simulink model "ssc_auto_ev_20b"  (R2020b)
settings: Solver=VariableStepAuto  StartTime=0.0  StopTime=200  RelTol=1e-3  AbsTol=1e-3
PreLoadFcn:
  | % Simulation parameters
  | dt = 0.01;
  | 
  | % Battery cell parameters
  | ssc_lithium_cell_1RC_ini
  | Nseries = 100;
  | Nparallel = 10;
  | 
  | % Motor parameters
  | max_torque = 220;
  | max_power = 80e3;
  | 
  | % Vehicle parameters
  | vehicle_mass = 4000;
  | wheel_radius = 0.35;
  | area = 5;
  | drag_coefficient = 0.25;
  | air_density = 1.225;
  | gravity = 9.81;
  | rolling_res_ratio = 0.015;
  | 
  | % Differential drive parameters
  | gear_ratio = 12;
  | 
  | % Simplified braking system parameters
  | force_max_pedal = 500;
  | braking_torque_to_pedal_force_ratio = -16;
  | 
  | % Vehicle controller parameters
  | hill_hold_max_speed = 0.5;
  | 
  | % Water properties for cooling circuit
  | load WaterProperties
  | 
  | % Input signals for Signal Editor block
  | load ssc_auto_ev_Inputs
values from neighbouring files (symbols this model uses):
  C1_LUT = [1913.6 4625.7 23306 10736 18036 12251 9022.9 12447 18872 40764 18721 33630 ... (21 elements, 7x3)]    [ssc_auto_ev_param.mat]
  Capacity_LUT = [28.0081 27.625 27.6392]    [ssc_auto_ev_param.mat]
  cell_Cp_heat = 810.5328    [ssc_auto_ev_param.mat]
  cell_mass = 1    [ssc_auto_ev_param.mat]
  Em_LUT = [3.4966 3.5519 3.6183 3.7066 3.9131 4.0748 4.1923 3.5057 3.566 3.6337 3.7127 3.9259 ... (21 elements, 7x3)]    [ssc_auto_ev_param.mat]
  Qe_init = 15.6845    [ssc_auto_ev_param.mat]
  R0_LUT = [0.0117 0.011 0.0114 0.0107 0.0107 0.0113 0.0116 0.0085 0.0085 0.0087 0.0082 0.0083 ... (21 elements, 7x3)]    [ssc_auto_ev_param.mat]
  R1_LUT = [0.0109 0.0069 0.0047 0.0034 0.0033 0.0033 0.0028 0.0029 0.0024 0.0026 0.0016 0.0023 ... (21 elements, 7x3)]    [ssc_auto_ev_param.mat]
  SOC_LUT = [0 0.1 0.25 0.5 0.75 0.9 1]    [ssc_auto_ev_param.mat]
  T_init = 293.15    [ssc_auto_ev_param.mat]
  Temperature_LUT = [278.15 293.15 313.15]    [ssc_auto_ev_param.mat]
undefined symbols (not defined in the file or in its folder): DiscIntNeverNeededParam, K, Lambda, tau, x0
libraries: fl_lib x656, nesl_utility x86, simulink x21, LiBatteryElements_lib x16, SignalEditorBlockLib x4, simulink_extras x4
(part 3 of 13)

== system ssc_auto_ev_20b/Step 4: Deployment Model ==
  note: Turn on sample time colors to validate timing. To do this, from the
      | DEBUG->DIAGNOSTICS menu select Information Overlays->Colors.
  Battery @50Hz : Subsystem
      settings: PortSchema="{\"entries\":[{\"content\":{\"sides\":[{\"content\":{\"connectorIds\":[\"In1\",\"Out2\"]},\"type\":\"ConnectorPlacement.EquallySpacedRectSide\",\"uuid\":\"54b288da-0e57-4d78-b35e-d63e4748356c\"},{\"content\":{\"connectorIds\":[\"Out1\",\"In2\"],\"side\":\"RIGHT\"},\"type\":\"ConnectorPlacement.EquallySpacedRectSide\",\"uuid\":\"06deb6c0-981d-4564-ae11-64776ad4ca27\"},{\"content\":{\"connectorIds\":[],\"side\":\"TOP\"},\"type\":\"ConnectorPlacement.EquallySpacedRectSide\",\"uuid\":\"0b8fba6d-2ee9-459b-aee7-2e2793598ae9\"}]},\"type\":\"ConnectorPlacement.EquallySpacedConnector\",\"uuid\":\"3f5b1629-deda-4b64-ac52-f3df4bebf2e4\"}],\"packageUris\":[\"http://schema.mathworks.com/mf0/Connector/R2020b\"],\"version\":\"1.0\"}"
  Control @100Hz : Subsystem
      settings: PortSchema="{\"entries\":[{\"content\":{\"sides\":[{\"content\":{\"connectorIds\":[]},\"type\":\"ConnectorPlacement.EquallySpacedRectSide\",\"uuid\":\"ef87f14a-ebef-48e8-8256-297aaa1e6a9a\"},{\"content\":{\"connectorIds\":[\"Out1\",\"In1\",\"Out2\",\"Out3\"],\"side\":\"RIGHT\"},\"type\":\"ConnectorPlacement.EquallySpacedRectSide\",\"uuid\":\"2f0c5370-6858-4894-ab47-0af24eaee6ce\"},{\"content\":{\"connectorIds\":[],\"side\":\"TOP\"},\"type\":\"ConnectorPlacement.EquallySpacedRectSide\",\"uuid\":\"12af46f8-0356-4b52-aec4-5ed7dbf12bbb\"}]},\"type\":\"ConnectorPlacement.EquallySpacedConnector\",\"uuid\":\"d882ff77-9b94-4690-a03a-88e1ef90f3db\"}],\"packageUris\":[\"http://schema.mathworks.com/mf0/Connector/R2020b\"],\"version\":\"1.0\"}"
  Rate Transition{,1..3} (4 alike) : RateTransition
  Rate transition (fast-to-slow){,1..3} (4 alike) : RateTransition  Integrity=off
  Rate transition (slow-to-fast){,1..3} (4 alike) : RateTransition  Integrity=off
  Thermal @20Hz : Subsystem
      settings: PortSchema="{\"entries\":[{\"content\":{\"sides\":[{\"content\":{\"connectorIds\":[\"In1\"]},\"type\":\"ConnectorPlacement.EquallySpacedRectSide\",\"uuid\":\"720b38ef-f1a9-4b25-942c-9d80c372deb3\"},{\"content\":{\"connectorIds\":[\"Out1\",\"In2\",\"Out2\",\"In3\",\"Out3\",\"In4\"],\"side\":\"RIGHT\"},\"type\":\"ConnectorPlacement.EquallySpacedRectSide\",\"uuid\":\"5564f5e5-3aff-4d95-92a7-b7874cc9818e\"},{\"content\":{\"connectorIds\":[],\"side\":\"TOP\"},\"type\":\"ConnectorPlacement.EquallySpacedRectSide\",\"uuid\":\"b2c1fdb5-3bc7-4a17-8874-08ad49945e58\"}]},\"type\":\"ConnectorPlacement.EquallySpacedConnector\",\"uuid\":\"56dd2a05-31e7-46fe-9962-826aaa21137d\"}],\"packageUris\":[\"http://schema.mathworks.com/mf0/Connector/R2020b\"],\"version\":\"1.0\"}"
  Vehicle and drive @100Hz : Subsystem
      settings: PortSchema="{\"entries\":[{\"content\":{\"sides\":[{\"content\":{\"connectorIds\":[\"In1\",\"Out1\",\"In2\",\"In3\",\"Out2\",\"In4\",\"Out3\",\"In5\",\"Out4\"]},\"type\":\"ConnectorPlacement.EquallySpacedRectSide\",\"uuid\":\"f314639a-2b4d-4845-a867-9fc19a275e88\"},{\"content\":{\"connectorIds\":[],\"side\":\"RIGHT\"},\"type\":\"ConnectorPlacement.EquallySpacedRectSide\",\"uuid\":\"94dc3db5-d98f-4c0a-adac-a7539403b4cc\"},{\"content\":{\"connectorIds\":[],\"side\":\"TOP\"},\"type\":\"ConnectorPlacement.EquallySpacedRectSide\",\"uuid\":\"a0a136c3-fb8b-4f8b-b3eb-c92638fab684\"}]},\"type\":\"ConnectorPlacement.EquallySpacedConnector\",\"uuid\":\"37a7cf0b-d138-4d1f-ae2f-6d44546dc5a7\"}],\"packageUris\":[\"http://schema.mathworks.com/mf0/Connector/R2020b\"],\"version\":\"1.0\"}"
  wires:
  Rate Transition/1 -> Thermal @20Hz/1(T)
  Rate transition (fast-to-slow)/1 -> Thermal @20Hz/2(temperature)
  Rate transition (fast-to-slow)2/1 -> Thermal @20Hz/3(temperature1)
  Rate transition (fast-to-slow)1/1 -> Thermal @20Hz/4(temperature2)
  Thermal @20Hz/1(heat flow) -> Rate transition (slow-to-fast)/1
  Thermal @20Hz/2(heat flow1) -> Rate transition (slow-to-fast)2/1
  Thermal @20Hz/3(heat flow2) -> Rate transition (slow-to-fast)1/1
  Rate transition (slow-to-fast)/1 -> Battery @50Hz/1(heat flow)
  Rate transition (fast-to-slow)3/1 -> Battery @50Hz/2(current)
  Battery @50Hz/1(voltage) -> Rate transition (slow-to-fast)3/1
  Battery @50Hz/2(temperature) -> Rate transition (fast-to-slow)/1
  Rate Transition2/1 -> Vehicle and drive @100Hz/1(Test data)
  Rate Transition1/1 -> Vehicle and drive @100Hz/2(iRef)
  Rate transition (slow-to-fast)3/1 -> Vehicle and drive @100Hz/3(voltage)
  Rate transition (slow-to-fast)2/1 -> Vehicle and drive @100Hz/4(heat flow)
  Rate transition (slow-to-fast)1/1 -> Vehicle and drive @100Hz/5(heat flow1)
  Vehicle and drive @100Hz/1(w) -> Rate Transition3/1
  Vehicle and drive @100Hz/2(current) -> Rate transition (fast-to-slow)3/1
  Vehicle and drive @100Hz/3(temperature) -> Rate transition (fast-to-slow)2/1
  Vehicle and drive @100Hz/4(temperature1) -> Rate transition (fast-to-slow)1/1
  Rate Transition3/1 -> Control @100Hz/1(In1)
  Control @100Hz/1(Veh) -> Rate Transition2/1
  Control @100Hz/2(Out2) -> Rate Transition1/1
  Control @100Hz/3(Env) -> Rate Transition/1

== system ssc_auto_ev_20b/Vehicle Dynamics ==
  Test data : Inport
  Brake Torque : Subsystem
  Bus Selector : BusSelector  OutputSignals=Incline,Wind speed,Brake pedal
  Drag and Gravity : Subsystem
  Final Drive Ratio : fl_lib/Mechanical/Mechanisms/Gear Box  ratio=gear_ratio  t_in_specify=off  t_in_priority=High  t_in=0 N*m  t_in_nominal_specify=off  t_in_nominal_unit=N*m  t_in_nominal_value=1  t_out_specify=off  t_out_priority=High  t_out=0 N*m  t_out_nominal_specify=off  t_out_nominal_unit=N*m  t_out_nominal_value=1
      settings: SourceProductBaseCode=PW,SS,VE
  Force Source : fl_lib/Mechanical/Mechanical Sources/Ideal Force Source
      settings: SourceProductBaseCode=PW,SS,VE
  MTRef : fl_lib/Mechanical/Translational Elements/Mechanical Translational Reference
      settings: SourceProductBaseCode=PW,SS,VE
  PS Subtract : fl_lib/Physical Signals/Functions/PS Subtract
      settings: SourceProductBaseCode=PW,SS,VE
  Sensing Speed : Subsystem
      mask Display: disp('v')
  Vehicle Mass : fl_lib/Mechanical/Translational Elements/Mass  mass=vehicle_mass kg  num_ports=foundation.enum.numPorts2.one  v_specify=off  v_priority=High  v=0 m/s  v_nominal_specify=off  v_nominal_unit=m/s  v_nominal_value=1  f_specify=off  f_priority=High  f=0 N  f_nominal_specify=off  f_nominal_unit=N  f_nominal_value=1
      settings: SourceProductBaseCode=PW,SS,VE
  Wheel and Axle : fl_lib/Mechanical/Mechanisms/Wheel and Axle  R=wheel_radius m  or=1  t_specify=off  t_priority=High  t=0 N*m  t_nominal_specify=off  t_nominal_unit=N*m  t_nominal_value=1  f_specify=off  f_priority=High  f=0 N  f_nominal_specify=off  f_nominal_unit=N  f_nominal_value=1
      settings: SourceProductBaseCode=PW,SS,VE
  R : PMIOPort  Side=Left
  wires:
  Bus Selector/2 -> Drag and Gravity/2(vW)  "<Wind speed>"
  Bus Selector/1 -> Drag and Gravity/1(beta)  "<Incline>"
  Bus Selector/3 -> Brake Torque/1(Pedal)  "<Brake pedal>"
  Test data/1 -> Bus Selector/1
  connections:
  Drag and Gravity/LConn1 -- Sensing Speed/RConn1
  Vehicle Mass/LConn1 -- Force Source/LConn1 -- Sensing Speed/LConn1 -- Wheel and Axle/RConn1
  Drag and Gravity/LConn2 -- PS Subtract/LConn2
  Drag and Gravity/LConn3 -- PS Subtract/LConn1
  PS Subtract/RConn1 -- Force Source/RConn1
  Wheel and Axle/LConn1 -- Final Drive Ratio/RConn1 -- Brake Torque/RConn1
  Force Source/RConn2 -- MTRef/LConn1
  R/RConn1 -- Final Drive Ratio/LConn1

== system ssc_auto_ev_20b/Vehicle Control ==
  ECU : Inport
  wMeas : Inport  Port=2
  -1 : Gain  Gain=-1
  1/Kt : Gain  Gain=1/1
  Bus Selector : BusSelector  OutputSignals=Cruise enable,Cruise disable,Brake pedal,Throttle,Incline
  Compare To Constant : simulink/Logic and Bit Operations/Compare To Constant  relop=>  const=0  OutDataTypeStr=boolean
  Cruise Control : Subsystem
  Feedforward term for regenerative braking on downhill : Subsystem
  Max Power : Subsystem
  Power limits : simulink/Discontinuities/Saturation Dynamic  OutMin=[]  OutMax=[]  OutDataTypeStr=Inherit: Same as second input  OutDataType=fixdt(1, 16)  OutScaling=2^-10  DoSatur=off
  Switch between torque control and speed control : Switch  Criteria=u2 > Threshold
  Torque limits : Saturate  UpperLimit=max_torque  LowerLimit=-max_torque
  Torque Demand Management : Subsystem
  iRef : Outport  VectorParamsAs1DForOutWhenUnconnected=off
  wires:
  Max Power/1(Max Power) -> Power limits/1, -1/1
  -1/1 -> Power limits/3
  Power limits/1 -> 1/Kt/1
  Torque limits/1 -> Power limits/2
  Bus Selector/5 -> Feedforward term for regenerative braking on downhill/1(Inclin.)  "<Incline>"
  Bus Selector/3 -> Compare To Constant/1, Torque Demand Management/1(Brake)  "<Brake pedal>"
  Bus Selector/4 -> Torque Demand Management/2(Throttle)  "<Throttle>"
  Compare To Constant/1 -> Cruise Control/4(Brake sw)
  Bus Selector/2 -> Cruise Control/2(Disable)  "<Cruise disable>"
  Cruise Control/1(trqRef) -> Switch between torque control and speed control/1
  wMeas/1 -> Torque Demand Management/3(wMeas), Cruise Control/3(wMeas), Max Power/1(Vspd)
  Bus Selector/1 -> Cruise Control/1(Enable)  "<Cruise enable>"
  Switch between torque control and speed control/1 -> Torque limits/1
  Torque Demand Management/1(Dem trq) -> Switch between torque control and speed control/3
  Cruise Control/2(Enabled) -> Switch between torque control and speed control/2
  ECU/1 -> Bus Selector/1
  1/Kt/1 -> iRef/1
  Feedforward term for regenerative braking on downhill/1(Feedfwd trq) -> Torque Demand Management/4(FFbrake)

== system ssc_auto_ev_20b/Battery/Electric and Thermal Model ==
  note: Equivalent Circuit Model for Single Battery Cell
  C1 : LiBatteryElements_lib/C_table  C_Table=C1_LUT*Nparallel F  SOC_Table=SOC_LUT  Temp_Table=Temperature_LUT K  v0=0 V
      settings: SourceProductBaseCode=SS  InternalSimscapePortConfiguration="{\"Bottom\":[],\"Left\":[{\"id\":\"p\",\"label\":\"+\",\"type\":\"foundation.electrical.electrical\"},{\"id\":\"T\",\"label\":\"T\",\"type\":\"input\"},{\"id\":\"SOC\",\"label\":\"SOC\",\"type\":\"input\"}],\"Right\":[{\"id\":\"n\",\"label\":\"-\",\"type\":\"foundation.electrical.electrical\"}],\"Top\":[]}"
  Em_table : LiBatteryElements_lib/Em_table  C_Table=Capacity_LUT*Nparallel hr*A  Em_Table=Em_LUT V  SOC_Table=SOC_LUT  Temp_Table=Temperature_LUT K  Qinit=Qe_init*Nparallel hr*A
      settings: SourceProductBaseCode=SS  InternalSimscapePortConfiguration="{\"Bottom\":[],\"Left\":[{\"id\":\"p\",\"label\":\"+\",\"type\":\"foundation.electrical.electrical\"},{\"id\":\"C\",\"label\":\"C\",\"type\":\"output\"},{\"id\":\"SOC\",\"label\":\"SOC\",\"type\":\"output\"}],\"Right\":[{\"id\":\"n\",\"label\":\"-\",\"type\":\"foundation.electrical.electrical\"},{\"id\":\"T\",\"label\":\"T\",\"type\":\"input\"}],\"Top\":[]}"
  NumCells : fl_lib/Physical Signals/Functions/PS Gain  gain=Nseries
      settings: SourceProductBaseCode=PW,SS,VE
  PS Add : fl_lib/Physical Signals/Functions/PS Add
      settings: SourceProductBaseCode=PW,SS,VE
  R0 : LiBatteryElements_lib/R_table  R_Table=R0_LUT/Nparallel Ohm  SOC_Table=SOC_LUT  Temp_Table=Temperature_LUT K
      settings: SourceProductBaseCode=SS  InternalSimscapePortConfiguration="{\"Bottom\":[],\"Left\":[{\"id\":\"p\",\"label\":\"+\",\"type\":\"foundation.electrical.electrical\"},{\"id\":\"T\",\"label\":\"T\",\"type\":\"input\"},{\"id\":\"SOC\",\"label\":\"SOC\",\"type\":\"input\"}],\"Right\":[{\"id\":\"n\",\"label\":\"-\",\"type\":\"foundation.electrical.electrical\"},{\"id\":\"pow\",\"label\":\"POW\",\"type\":\"output\"}],\"Top\":[]}"
  R1 : LiBatteryElements_lib/R_table  R_Table=R1_LUT/Nparallel Ohm  SOC_Table=SOC_LUT  Temp_Table=Temperature_LUT K
      settings: SourceProductBaseCode=SS  InternalSimscapePortConfiguration="{\"Bottom\":[],\"Left\":[{\"id\":\"p\",\"label\":\"+\",\"type\":\"foundation.electrical.electrical\"},{\"id\":\"T\",\"label\":\"T\",\"type\":\"input\"},{\"id\":\"SOC\",\"label\":\"SOC\",\"type\":\"input\"}],\"Right\":[{\"id\":\"n\",\"label\":\"-\",\"type\":\"foundation.electrical.electrical\"},{\"id\":\"pow\",\"label\":\"POW\",\"type\":\"output\"}],\"Top\":[]}"
  Thermal Model : Subsystem
  + : PMIOPort  Side=Right
  - : PMIOPort  Port=2  Side=Right
  H : PMIOPort  Tag=PMCPort  Port=3  Side=Left
  connections:
  H/RConn1 -- Thermal Model/LConn2
  NumCells/RConn1 -- Thermal Model/LConn1
  R1/LConn3 -- C1/LConn3 -- Em_table/LConn3 -- R0/LConn3
  Em_table/RConn1 -- -/RConn1
  R0/LConn1 -- R1/RConn1 -- C1/RConn1
  PS Add/LConn1 -- R0/RConn2
  PS Add/LConn2 -- R1/RConn2
  C1/LConn1 -- R1/LConn1 -- Em_table/LConn1
  R1/LConn2 -- Thermal Model/RConn1 -- Em_table/RConn2 -- R0/LConn2 -- C1/LConn2
  +/RConn1 -- R0/RConn1
  PS Add/RConn1 -- NumCells/LConn1

== system ssc_auto_ev_20b/Cooling System/ Heat Exchanger Characteristic ==
  Characteristic : Subsystem
  Heat Flow Source : fl_lib/Thermal/Thermal Sources/Controlled Heat Flow Rate Source
      settings: SourceProductBaseCode=PW,SS,VE
  Mass Flow Rate & Thermal Flux Sensor (TL) : fl_lib/Thermal Liquid/Sensors/Mass & Energy Flow Rate Sensor (TL)
      settings: SourceProductBaseCode=PW,SS,VE  InternalSimscapePortConfiguration="{\"Bottom\":[],\"Left\":[{\"id\":\"A\",\"label\":\"A\",\"type\":\"foundation.thermal_liquid.thermal_liquid\"}],\"Right\":[{\"id\":\"B\",\"label\":\"B\",\"type\":\"foundation.thermal_liquid.thermal_liquid\"},{\"id\":\"M\",\"label\":\"M\",\"type\":\"output\"},{\"id\":\"PHI\",\"label\":\"Phi\",\"type\":\"output\"}],\"Top\":[]}"
  Temperature Sensor : fl_lib/Thermal/Thermal Sensors/Temperature Sensor
      settings: SourceProductBaseCode=PW,SS,VE
  ThRef : fl_lib/Thermal/Thermal Elements/Thermal Reference
      settings: SourceProductBaseCode=PW,SS,VE
  Henv : PMIOPort  Side=Right
  Hp : PMIOPort  Port=2  Side=Left
  B : PMIOPort  Port=3  Side=Right
  Phi : PMIOPort  Port=4  Side=Right
  A : PMIOPort  Port=5  Side=Left
  T in : PMIOPort  Port=6  Side=Left
  connections:
  Characteristic/LConn1 -- Heat Flow Source/RConn1
  Temperature Sensor/RConn2 -- Characteristic/RConn3
  T in/RConn1 -- Characteristic/RConn2
  Mass Flow Rate & Thermal Flux Sensor (TL)/RConn2 -- Characteristic/RConn1
  Mass Flow Rate & Thermal Flux Sensor (TL)/RConn3 -- Phi/RConn1
  Mass Flow Rate & Thermal Flux Sensor (TL)/RConn1 -- B/RConn1
  Heat Flow Source/LConn1 -- Hp/RConn1
  ThRef/LConn1 -- Temperature Sensor/RConn1
  Heat Flow Source/RConn2 -- Henv/RConn1 -- Temperature Sensor/LConn1
  A/RConn1 -- Mass Flow Rate & Thermal Flux Sensor (TL)/LConn1

== system ssc_auto_ev_20b/Cooling System/Expansion Tank ==
  Air Stiffness : fl_lib/Mechanical/Translational Elements/Translational Spring  spr_rate=1e3 N/m  v_specify=off  v_priority=High  v=0 m/s  v_nominal_specify=off  v_nominal_unit=m/s  v_nominal_value=1  f_specify=on  f_priority=Low  f=0 N  f_nominal_specify=off  f_nominal_unit=N  f_nominal_value=1  x_specify=off  x_priority=High  x=0 m  x_nominal_specify=off  x_nominal_unit=m  x_nominal_value=1
      settings: SourceProductBaseCode=PW,SS,VE
  Expansion Tank : fl_lib/Thermal Liquid/Elements/Translational Mechanical Converter (TL)  mech_orientation=1  interface_area=pi*50^2 mm^2  x0=200 mm  dead_volume=0.001 m^3  environment_spec=1  environment_pressure=0.101325 MPa  dynamic_compressibility=0  p0=1 atm  T0=20 degC
      settings: SourceProductBaseCode=PW,SS,VE  InternalSimscapePortConfiguration="{\"Bottom\":[],\"Left\":[{\"id\":\"A\",\"label\":\"A\",\"type\":\"foundation.thermal_liquid.thermal_liquid\"},{\"id\":\"C\",\"label\":\"C\",\"type\":\"foundation.mechanical.translational.translational\"},{\"id\":\"H\",\"label\":\"H\",\"type\":\"foundation.thermal.thermal\"}],\"Right\":[{\"id\":\"R\",\"label\":\"R\",\"type\":\"foundation.mechanical.translational.translational\"}],\"Top\":[]}"
  Expansion Tank Inlet : fl_lib/Thermal Liquid/Elements/Local Restriction (TL)  restriction_type=foundation.enum.restriction_type.fixed  restriction_area=pi*10^2 mm^2  min_area=1e-10 m^2  max_area=0.005 m^2  area=pi*11^2 mm^2  Cd=0.7  pressure_recovery=0  Re_c=12
      settings: SourceProductBaseCode=PW,SS,VE
  Insulator Expansion Tank : fl_lib/Thermal/Thermal Elements/Perfect Insulator  T_specify=off  T_priority=High  T=0 K  T_nominal_specify=off  T_nominal_unit=K  T_nominal_value=1
      settings: SourceProductBaseCode=PW,SS,VE
  MTRef : fl_lib/Mechanical/Translational Elements/Mechanical Translational Reference
      settings: SourceProductBaseCode=PW,SS,VE
  MTRef Air Stiffness : fl_lib/Mechanical/Translational Elements/Mechanical Translational Reference
      settings: SourceProductBaseCode=PW,SS,VE
  A : PMIOPort  Side=Left
  connections:
  MTRef/LConn1 -- Expansion Tank/LConn2
  Insulator Expansion Tank/LConn1 -- Expansion Tank/LConn3
  Expansion Tank Inlet/LConn1 -- A/RConn1
  Expansion Tank Inlet/RConn1 -- Expansion Tank/LConn1
  Air Stiffness/LConn1 -- Expansion Tank/RConn1
  Air Stiffness/RConn1 -- MTRef Air Stiffness/LConn1

== system ssc_auto_ev_20b/Cooling System/Heat Exchanger Characteristic ==
  Characteristic : Subsystem
  Heat Flow Source : fl_lib/Thermal/Thermal Sources/Controlled Heat Flow Rate Source
      settings: SourceProductBaseCode=PW,SS,VE
  Mass Flow Rate & Thermal Flux Sensor (TL) : fl_lib/Thermal Liquid/Sensors/Mass & Energy Flow Rate Sensor (TL)
      settings: SourceProductBaseCode=PW,SS,VE  InternalSimscapePortConfiguration="{\"Bottom\":[],\"Left\":[{\"id\":\"A\",\"label\":\"A\",\"type\":\"foundation.thermal_liquid.thermal_liquid\"}],\"Right\":[{\"id\":\"B\",\"label\":\"B\",\"type\":\"foundation.thermal_liquid.thermal_liquid\"},{\"id\":\"M\",\"label\":\"M\",\"type\":\"output\"},{\"id\":\"PHI\",\"label\":\"Phi\",\"type\":\"output\"}],\"Top\":[]}"
  Temperature Sensor : fl_lib/Thermal/Thermal Sensors/Temperature Sensor
      settings: SourceProductBaseCode=PW,SS,VE
  ThRef : fl_lib/Thermal/Thermal Elements/Thermal Reference
      settings: SourceProductBaseCode=PW,SS,VE
  HMotor : PMIOPort  Side=Right
  B : PMIOPort  Port=2  Side=Right
  Hp : PMIOPort  Port=3  Side=Left
  A : PMIOPort  Port=4  Side=Left
  TIn : PMIOPort  Port=5  Side=Left
  connections:
  Characteristic/RConn1 -- Heat Flow Source/RConn1
  Characteristic/LConn2 -- TIn/RConn1
  Mass Flow Rate & Thermal Flux Sensor (TL)/RConn2 -- Characteristic/LConn1
  Temperature Sensor/RConn2 -- Characteristic/LConn3
  A/RConn1 -- Mass Flow Rate & Thermal Flux Sensor (TL)/LConn1
  Heat Flow Source/LConn1 -- Hp/RConn1
  ThRef/LConn1 -- Temperature Sensor/RConn1
  HMotor/RConn1 -- Temperature Sensor/LConn1 -- Heat Flow Source/RConn2
  Mass Flow Rate & Thermal Flux Sensor (TL)/RConn1 -- B/RConn1

== system ssc_auto_ev_20b/Cooling System/Sensing Inlet Temperature ==
  Pressure & Temperature Sensor (TL) : fl_lib/Thermal Liquid/Sensors/Pressure & Temperature Sensor (TL)
      settings: SourceProductBaseCode=PW,SS,VE  InternalSimscapePortConfiguration="{\"Bottom\":[],\"Left\":[{\"id\":\"A\",\"label\":\"A\",\"type\":\"foundation.thermal_liquid.thermal_liquid\"}],\"Right\":[{\"id\":\"B\",\"label\":\"B\",\"type\":\"foundation.thermal_liquid.thermal_liquid\"},{\"id\":\"P\",\"label\":\"P\",\"type\":\"output\"},{\"id\":\"T\",\"label\":\"T\",\"type\":\"output\"}],\"Top\":[]}"
  TLRef : fl_lib/Thermal Liquid/Elements/Absolute Reference (TL)
      settings: SourceProductBaseCode=PW,SS,VE
  A : PMIOPort  Side=Left
  T : PMIOPort  Port=2  Side=Right
  connections:
  TLRef/LConn1 -- Pressure & Temperature Sensor (TL)/RConn1
  Pressure & Temperature Sensor (TL)/LConn1 -- A/RConn1
  Pressure & Temperature Sensor (TL)/RConn3 -- T/RConn1

== system ssc_auto_ev_20b/Cooling System/Sensing Temperature ==
  Pressure & Temperature Sensor (TL) : fl_lib/Thermal Liquid/Sensors/Pressure & Temperature Sensor (TL)
      settings: SourceProductBaseCode=PW,SS,VE  InternalSimscapePortConfiguration="{\"Bottom\":[],\"Left\":[{\"id\":\"A\",\"label\":\"A\",\"type\":\"foundation.thermal_liquid.thermal_liquid\"}],\"Right\":[{\"id\":\"B\",\"label\":\"B\",\"type\":\"foundation.thermal_liquid.thermal_liquid\"},{\"id\":\"P\",\"label\":\"P\",\"type\":\"output\"},{\"id\":\"T\",\"label\":\"T\",\"type\":\"output\"}],\"Top\":[]}"
  TLRef : fl_lib/Thermal Liquid/Elements/Absolute Reference (TL)
      settings: SourceProductBaseCode=PW,SS,VE
  T : PMIOPort  Side=Right
  A : PMIOPort  Port=2  Side=Left
  connections:
  A/RConn1 -- Pressure & Temperature Sensor (TL)/LConn1
  TLRef/LConn1 -- Pressure & Temperature Sensor (TL)/RConn1
  Pressure & Temperature Sensor (TL)/RConn3 -- T/RConn1

== system ssc_auto_ev_20b/Driver and Environment/Bus ==
  In : Inport
  Wi : Inport  Port=2
  Br : Inport  Port=3
  Bus Creator : BusCreator  Inputs=3
  b : Outport  VectorParamsAs1DForOutWhenUnconnected=off
  wires:
  In/1 -> Bus Creator/1  "Incline"
  Br/1 -> Bus Creator/3  "Brake pedal"
  Bus Creator/1 -> b/1
  Wi/1 -> Bus Creator/2  "Wind speed"

== system ssc_auto_ev_20b/Driver and Environment/Inclinometer ==
  a : Inport
  Trigonometric Function : Trigonometry
  d2r : Gain  Gain=pi/180
  g : Gain  Gain=gravity
  y : Outport  VectorParamsAs1DForOutWhenUnconnected=off
  wires:
  g/1 -> y/1
  d2r/1 -> Trigonometric Function/1
  a/1 -> d2r/1
  Trigonometric Function/1 -> g/1

== system ssc_auto_ev_20b/Motor Drive/DC Motor1 ==
  Inertia : fl_lib/Mechanical/Rotational Elements/Inertia  inertia=0.01 kg*m^2  num_ports=foundation.enum.numPorts2.one  w_specify=off  w_priority=High  w=0 rad/s  w_nominal_specify=off  w_nominal_unit=rad/s  w_nominal_value=1  t_specify=off  t_priority=High  t=0 N*m  t_nominal_specify=off  t_nominal_unit=N*m  t_nominal_value=1
      settings: SourceProductBaseCode=PW,SS,VE
  Rotational Electromechanical Converter : fl_lib/Electrical/Electrical Elements/Rotational Electromechanical Converter  K=1 N*m/A  i_specify=off  i_priority=High  i=0 A  i_nominal_specify=off  i_nominal_unit=A  i_nominal_value=1  v_specify=off  v_priority=High  v=0 V  v_nominal_specify=off  v_nominal_unit=V  v_nominal_value=1  t_specify=off  t_priority=High  t=0 N*m  t_nominal_specify=off  t_nominal_unit=N*m  t_nominal_value=1  w_specify=off  w_priority=High  w=0 rad/s  w_nominal_specify=off  w_nominal_unit=rad/s  w_nominal_value=1
      settings: SourceProductBaseCode=PW,SS,VE
  Thermal Resistor : fl_lib/Electrical/Electrical Elements/Thermal Resistor  R0=1 Ohm  T0=298.15 K  alpha=50e-6 1/K  tc=30 s  K_d=100 W/K  T_specify=off  T_priority=High  T=300 K  T_nominal_specify=off  T_nominal_unit=K  T_nominal_value=1
      settings: SourceProductBaseCode=PW,SS,VE  InternalSimscapePortConfiguration="{\"Bottom\":[],\"Left\":[{\"id\":\"H\",\"label\":\"H\",\"type\":\"foundation.thermal.thermal\"},{\"id\":\"p\",\"label\":\"+\",\"type\":\"foundation.electrical.electrical\"}],\"Right\":[{\"id\":\"n\",\"label\":\"-\",\"type\":\"foundation.electrical.electrical\"}],\"Top\":[]}"
  V+ : PMIOPort  Side=Left
  R : PMIOPort  Port=2  Side=Right
  C : PMIOPort  Port=3  Side=Right
  V- : PMIOPort  Port=4  Side=Left
  H : PMIOPort  Port=5  Side=Left
  connections:
  V-/RConn1 -- Rotational Electromechanical Converter/RConn1
  Thermal Resistor/LConn2 -- V+/RConn1
  Rotational Electromechanical Converter/LConn1 -- Thermal Resistor/RConn1
  Rotational Electromechanical Converter/LConn2 -- Inertia/LConn1 -- R/RConn1
  Rotational Electromechanical Converter/RConn2 -- C/RConn1
  H/RConn1 -- Thermal Resistor/LConn1

== system ssc_auto_ev_20b/Motor Drive/DC Motor2 ==
  Inertia : fl_lib/Mechanical/Rotational Elements/Inertia  inertia=0.01 kg*m^2  num_ports=foundation.enum.numPorts2.one  w_specify=off  w_priority=High  w=0 rad/s  w_nominal_specify=off  w_nominal_unit=rad/s  w_nominal_value=1  t_specify=off  t_priority=High  t=0 N*m  t_nominal_specify=off  t_nominal_unit=N*m  t_nominal_value=1
      settings: SourceProductBaseCode=PW,SS,VE
  Rotational Electromechanical Converter : fl_lib/Electrical/Electrical Elements/Rotational Electromechanical Converter  K=1 N*m/A  i_specify=off  i_priority=High  i=0 A  i_nominal_specify=off  i_nominal_unit=A  i_nominal_value=1  v_specify=off  v_priority=High  v=0 V  v_nominal_specify=off  v_nominal_unit=V  v_nominal_value=1  t_specify=off  t_priority=High  t=0 N*m  t_nominal_specify=off  t_nominal_unit=N*m  t_nominal_value=1  w_specify=off  w_priority=High  w=0 rad/s  w_nominal_specify=off  w_nominal_unit=rad/s  w_nominal_value=1
      settings: SourceProductBaseCode=PW,SS,VE
  Thermal Resistor : fl_lib/Electrical/Electrical Elements/Thermal Resistor  R0=1 Ohm  T0=298.15 K  alpha=50e-6 1/K  tc=30 s  K_d=100 W/K  T_specify=off  T_priority=High  T=300 K  T_nominal_specify=off  T_nominal_unit=K  T_nominal_value=1
      settings: SourceProductBaseCode=PW,SS,VE  InternalSimscapePortConfiguration="{\"Bottom\":[],\"Left\":[{\"id\":\"H\",\"label\":\"H\",\"type\":\"foundation.thermal.thermal\"},{\"id\":\"p\",\"label\":\"+\",\"type\":\"foundation.electrical.electrical\"}],\"Right\":[{\"id\":\"n\",\"label\":\"-\",\"type\":\"foundation.electrical.electrical\"}],\"Top\":[]}"
  V+ : PMIOPort  Side=Left
  R : PMIOPort  Port=2  Side=Right
  C : PMIOPort  Port=3  Side=Right
  V- : PMIOPort  Port=4  Side=Left
  H : PMIOPort  Port=5  Side=Left
  connections:
  H/RConn1 -- Thermal Resistor/LConn1
  Rotational Electromechanical Converter/RConn2 -- C/RConn1
  R/RConn1 -- Inertia/LConn1 -- Rotational Electromechanical Converter/LConn2
  Thermal Resistor/LConn2 -- V+/RConn1
  V-/RConn1 -- Rotational Electromechanical Converter/RConn1
  Thermal Resistor/RConn1 -- Rotational Electromechanical Converter/LConn1

== system ssc_auto_ev_20b/Motor Drive/Motor Torque Controller 1 (System-Level Representation) ==
  Controlled Current Source : fl_lib/Electrical/Electrical Sources/Controlled Current Source
      settings: SourceProductBaseCode=PW,SS,VE
  +1 : PMIOPort  Side=Right
  +2 : PMIOPort  Port=2  Side=Left
  -1 : PMIOPort  Port=3  Side=Right
  -2 : PMIOPort  Port=4  Side=Left
  iRef : PMIOPort  Port=5  Side=Left
  connections:
  Controlled Current Source/RConn2 -- +1/RConn1
  Controlled Current Source/LConn1 -- +2/RConn1
  -2/RConn1 -- -1/RConn1
  iRef/RConn1 -- Controlled Current Source/RConn1

== system ssc_auto_ev_20b/Motor Drive/Motor Torque Controller 1 (System-Level Representation)1 ==
  Controlled Current Source : fl_lib/Electrical/Electrical Sources/Controlled Current Source
      settings: SourceProductBaseCode=PW,SS,VE
  +1 : PMIOPort  Side=Right
  +2 : PMIOPort  Port=2  Side=Left
  -1 : PMIOPort  Port=3  Side=Right
  -2 : PMIOPort  Port=4  Side=Left
  iRef : PMIOPort  Port=5  Side=Left
  connections:
  iRef/RConn1 -- Controlled Current Source/RConn1
  -2/RConn1 -- -1/RConn1
  Controlled Current Source/LConn1 -- +2/RConn1
  Controlled Current Source/RConn2 -- +1/RConn1

== system ssc_auto_ev_20b/Motor Drive/Sensing wMotor ==
  PS-Simulink Converter : nesl_utility/PS-Simulink Converter  PhysicalDomain=network_engine_domain  SubClassName=ps_output  LeftPortType=input  RightPortType=output  PseudoPeriodic=off  Frequencies=[]  Unit=rad/s  AffineConversion=off
      settings: SourceProductBaseCode=SS,PW,VE
  PS : PMIOPort  Side=Left
  SL : Outport  VectorParamsAs1DForOutWhenUnconnected=off
  wires:
  PS-Simulink Converter/1 -> SL/1
  connections:
  PS/RConn1 -- PS-Simulink Converter/LConn1

== system ssc_auto_ev_20b/Step 2: Multirate Model/Battery ==
  note: Scale up voltage drop to total
      | of Ns series-connected cells
  Controlled Voltage Source : fl_lib/Electrical/Electrical Sources/Controlled Voltage Source
      settings: SourceProductBaseCode=PW,SS,VE
  Electric and Thermal Model : Subsystem  Tag=PublishSubsystem
  Nseries-1 : fl_lib/Physical Signals/Functions/PS Gain  gain=Nseries-1
      settings: SourceProductBaseCode=PW,SS,VE
  PS Terminator : fl_lib/Physical Signals/Sinks/PS Terminator
      settings: SourceProductBaseCode=PW,SS,VE
  Temperature Sensor : fl_lib/Thermal/Thermal Sensors/Temperature Sensor
      settings: SourceProductBaseCode=PW,SS,VE
  Thermal Reference : fl_lib/Thermal/Thermal Elements/Thermal Reference
      settings: SourceProductBaseCode=PW,SS,VE
  Voltage Sensor : fl_lib/Electrical/Electrical Sensors/Voltage Sensor
      settings: SourceProductBaseCode=PW,SS,VE
  + : PMIOPort  Tag=PMCPort  Side=Right
  H : PMIOPort  Tag=PMCPort  Port=2  Side=Left
  - : PMIOPort  Tag=PMCPort  Port=3  Side=Left
  connections:
  H/RConn1 -- Temperature Sensor/LConn1 -- Electric and Thermal Model/LConn1
  Controlled Voltage Source/LConn1 -- Voltage Sensor/RConn2 -- Electric and Thermal Model/RConn2
  Nseries-1/LConn1 -- Voltage Sensor/RConn1
  Voltage Sensor/LConn1 -- Electric and Thermal Model/RConn1 -- +/RConn1
  Nseries-1/RConn1 -- Controlled Voltage Source/RConn1
  Controlled Voltage Source/RConn2 -- -/RConn1
  Temperature Sensor/RConn1 -- Thermal Reference/LConn1
  PS Terminator/LConn1 -- Temperature Sensor/RConn2

== system ssc_auto_ev_20b/Step 2: Multirate Model/Battery Thermal Mass ==
  note: Connect Port 1 to the network
      | with the smaller sample time, or
      | the network running variable step.
  note: Uncomment rate transition
      | blocks if one or both networks
      | are running fixed step.
  Port 1 Interface : Subsystem  mask(Network Coupler (Thermal Mass) Port 1 Interface){thermalMass=cell_mass*Nseries*Nparallel*cell_Cp_heat, samplingType=physmod:simscape:couplers:SimscapeNetworkCouplersLib:VariableStepAtPorts1And2_PV, h1=dt*2, h2=dt*5, predictionDiscreteToContinuous=off, smoothingContinuousToDiscrete=off, predictionSlowToFast=off, smoothingFastToSlow=off, nSmooth=1, tsSmoothing=0.01, thermalConductanceNetwork=1, hRecommended=0.001, T0=T_init}
      mask prompts: thermalMass "physmod:simscape:couplers:SimscapeNetworkCouplersLib:ThermalMassJK_MP"; samplingType "physmod:simscape:couplers:SimscapeNetworkCouplersLib:SamplingType_MP"; h1 "physmod:simscape:couplers:SimscapeNetworkCouplersLib:Port1NetworkDiscreteSampleTimes_MP"; h2 "physmod:simscape:couplers:SimscapeNetworkCouplersLib:Port2NetworkDiscreteSampleTimes_MP"; predictionDiscreteToContinuous "physmod:simscape:couplers:SimscapeNetworkCouplersLib:UsePredictionWhenConnectingFixedStepToVariableStep_MP"; smoothingContinuousToDiscrete "physmod:simscape:couplers:SimscapeNetworkCouplersLib:UseSmoothingWhenConnectingVariableStepToFixedStep_MP"; predictionSlowToFast "physmod:simscape:couplers:SimscapeNetworkCouplersLib:UsePredictionWhenConnectingSlowToFastSampleTimes_MP"; smoothingFastToSlow "physmod:simscape:couplers:SimscapeNetworkCouplersLib:UseSmoothingWhenConnectingFastToSlowSampleTimes_MP"; nSmooth "physmod:simscape:couplers:SimscapeNetworkCouplersLib:NumberOfSamplesOverWhichToSmooth_MP"; tsSmoothing "physmod:simscape:couplers:SimscapeNetworkCouplersLib:SmoothingTimeConstants_MP"; thermalConductanceNetwork "physmod:simscape:couplers:SimscapeNetworkCouplersLib:ApproximateConnectedNetworkThermalConductanceWK_MP"; hRecommended "physmod:simscape:couplers:SimscapeNetworkCouplersLib:RecommendedMaxDiscreteSampleTimes_MP"; T0 "physmod:simscape:couplers:SimscapeNetworkCouplersLib:InitialTemperatureK_MP"
      mask help: physmod:simscape:couplers:SimscapeNetworkCouplersLib:NetworkCouplerThermalMassPort1Interface_MD
      mask init: same as ssc_auto_ev_20b/Step 3: Ungroup and Redraw/Port 1 Interface1
      settings: PortSchema="{\"entries\":[{\"content\":{\"sides\":[{\"content\":{\"connectorIds\":[\"LConn1\"]},\"type\":\"ConnectorPlacement.EquallySpacedRectSide\",\"uuid\":\"a6d4a9fd-b5aa-40dc-ab7e-2b646b9b57bc\"},{\"content\":{\"connectorIds\":[\"Out1\",\"In1\"],\"side\":\"RIGHT\"},\"type\":\"ConnectorPlacement.EquallySpacedRectSide\",\"uuid\":\"31bb6273-5b9b-48d0-a1a2-6fbacb979b97\"},{\"content\":{\"connectorIds\":[],\"side\":\"TOP\"},\"type\":\"ConnectorPlacement.EquallySpacedRectSide\",\"uuid\":\"0f7afab2-4481-486c-9ad0-2b42c5b091a4\"}]},\"type\":\"ConnectorPlacement.EquallySpacedConnector\",\"uuid\":\"a98e47aa-cbfd-441a-b14c-c9ea515c056e\"}],\"packageUris\":[\"http://schema.mathworks.com/mf0/Connector/R2020b\"],\"version\":\"1.0\"}"
      mask Help: web([docroot '/physmod/simscape/ref/networkcouplerthermalmass.html'])
      mask TypeOptions samplingType: physmod:simscape:couplers:SimscapeNetworkCouplersLib:VariableStepAtPorts1And2_PV | physmod:simscape:couplers:SimscapeNetworkCouplersLib:VariableStepAtPort1AndFixedStepAtPort2_PV | physmod:simscape:couplers:SimscapeNetworkCouplersLib:FixedStepBothPortsWithCommonSampleTime_PV | physmod:simscape:couplers:SimscapeNetworkCouplersLib:FixedStepBothPortsWithFasterSamplingAtPort1_PV
      mask Callback samplingType: foundation.internal.couplers.thermal.parameterVisibilitiesThermalMass(gcb)
      mask Callback predictionDiscreteToContinuous: foundation.internal.couplers.thermal.parameterVisibilitiesThermalMass(gcb)
      mask Callback smoothingContinuousToDiscrete: foundation.internal.couplers.thermal.parameterVisibilitiesThermalMass(gcb)
      mask Callback predictionSlowToFast: foundation.internal.couplers.thermal.parameterVisibilitiesThermalMass(gcb)
      mask Callback smoothingFastToSlow: foundation.internal.couplers.thermal.parameterVisibilitiesThermalMass(gcb)
      mask DialogControl Main Prompt: Main
      mask DialogControl Analysis Prompt: Analysis
      mask DialogControl connectedNetworkInfo Prompt: Connected network information
      mask DialogControl derivedValues Prompt: Derived values
      mask DialogControl updateRecommendations Prompt: Update
      mask DialogControl updateRecommendations Callback: foundation.internal.couplers.thermal.analysisThermalMass(gcb);
      mask DialogControl InitialConditions Prompt: Initial Conditions
  Port 2 Interface : Subsystem  mask(Network Coupler (Thermal Mass) Port 2 Interface){}
      mask help: physmod:simscape:couplers:SimscapeNetworkCouplersLib:NetworkCouplerThermalMassPort2Interface_MD
      settings: PortSchema="{\"entries\":[{\"content\":{\"sides\":[{\"content\":{\"connectorIds\":[\"In1\",\"Out1\"]},\"type\":\"ConnectorPlacement.EquallySpacedRectSide\",\"uuid\":\"5a4c1550-e77d-42df-bf3e-b81963920de7\"},{\"content\":{\"connectorIds\":[\"RConn1\"],\"side\":\"RIGHT\"},\"type\":\"ConnectorPlacement.EquallySpacedRectSide\",\"uuid\":\"3fd730f7-5937-4563-a365-595aaae9027b\"},{\"content\":{\"connectorIds\":[],\"side\":\"TOP\"},\"type\":\"ConnectorPlacement.EquallySpacedRectSide\",\"uuid\":\"c16e04e4-26e8-4fd6-98d3-59adbef44c0d\"}]},\"type\":\"ConnectorPlacement.EquallySpacedConnector\",\"uuid\":\"5588d8d0-d459-45fe-a303-1ca6654e99d0\"}],\"packageUris\":[\"http://schema.mathworks.com/mf0/Connector/R2020b\"],\"version\":\"1.0\"}"
      mask Help: web([docroot '/physmod/simscape/ref/networkcouplerthermalmass.html'])
  Rate transition (fast-to-slow) : RateTransition  Integrity=off
  Rate transition (slow-to-fast) : RateTransition  Integrity=off
  1 : PMIOPort  Side=Left
  2 : PMIOPort  Port=2  Side=Right
  wires:
  Rate transition (slow-to-fast)/1 -> Port 1 Interface/1(heat flow)
  Port 2 Interface/1(heat flow) -> Rate transition (slow-to-fast)/1
  Rate transition (fast-to-slow)/1 -> Port 2 Interface/1(temperature)
  Port 1 Interface/1(temperature) -> Rate transition (fast-to-slow)/1
  connections:
  1/RConn1 -- Port 1 Interface/LConn1
  2/RConn1 -- Port 2 Interface/RConn1

== system ssc_auto_ev_20b/Step 2: Multirate Model/Cooling System ==
  note: Radiator
  note: Battery Heat Exchanger
  " Heat Exchanger Characteristic" : Subsystem
  Convection Battery-Env : fl_lib/Thermal/Thermal Elements/Convective Heat Transfer  area=cell_area m^2  heat_tr_coeff=h_conv W/(m^2 * K)  T_specify=off  T_priority=High  T=0 K  T_nominal_specify=off  T_nominal_unit=K  T_nominal_value=1  Q_specify=off  Q_priority=High  Q=0 J/s  Q_nominal_specify=off  Q_nominal_unit=J/s  Q_nominal_value=1
      settings: SourceProductBaseCode=PW,SS,VE
  Expansion Tank : Subsystem
  Heat Exchanger Characteristic : Subsystem
  Hose Radiator : fl_lib/Thermal Liquid/Elements/Pipe (TL)  length=2000 mm  area=pi*25^2 mm^2  Dh=50 mm  length_add=500 mm  roughness=1.5e-5 m  Re_lam=2e+3  Re_tur=4e+3  shape_factor=64  Nu_lam=3.66  dynamic_compressibility=1  inertia=0  p0=1 atm  T0=20 degC  mdot0=0.1 kg/s
      settings: SourceProductBaseCode=PW,SS,VE
  Hose Inlet : fl_lib/Thermal Liquid/Elements/Pipe (TL)  length=500 mm  area=pi*25^2 mm^2  Dh=50 mm  length_add=500 mm  roughness=1.5e-5 m  Re_lam=2e+3  Re_tur=4e+3  shape_factor=64  Nu_lam=3.66  dynamic_compressibility=1  inertia=0  p0=1 atm  T0=20 degC  mdot0=0.1 kg/s
      settings: SourceProductBaseCode=PW,SS,VE
  Hose Outlet : fl_lib/Thermal Liquid/Elements/Pipe (TL)  length=500 mm  area=pi*25^2 mm^2  Dh=50 mm  length_add=500 mm  roughness=1.5e-5 m  Re_lam=2e+3  Re_tur=4e+3  shape_factor=64  Nu_lam=3.66  dynamic_compressibility=1  inertia=0  p0=1 atm  T0=20 degC  mdot0=0.1 kg/s
      settings: SourceProductBaseCode=PW,SS,VE
  Insulator Inlet Hose : fl_lib/Thermal/Thermal Elements/Perfect Insulator  T_specify=off  T_priority=High  T=0 K  T_nominal_specify=off  T_nominal_unit=K  T_nominal_value=1
      settings: SourceProductBaseCode=PW,SS,VE
  Insulator Outlet Hose : fl_lib/Thermal/Thermal Elements/Perfect Insulator  T_specify=off  T_priority=High  T=0 K  T_nominal_specify=off  T_nominal_unit=K  T_nominal_value=1
      settings: SourceProductBaseCode=PW,SS,VE
  PS Terminator : fl_lib/Physical Signals/Sinks/PS Terminator
      settings: SourceProductBaseCode=PW,SS,VE
  Pipe : fl_lib/Thermal Liquid/Elements/Pipe (TL)  length=400 mm  area=pi*25^2 mm^2  Dh=50 mm  length_add=500 mm  roughness=1.5e-5 m  Re_lam=2e+3  Re_tur=4e+3  shape_factor=64  Nu_lam=3.66  dynamic_compressibility=1  inertia=0  p0=1 atm  T0=20 degC  mdot0=0.1 kg/s
      settings: SourceProductBaseCode=PW,SS,VE
  Pump : fl_lib/Thermal Liquid/Sources/Mass Flow Rate Source (TL)  commanded_mass_flow=0.2 kg/s  area=pi*25^2 mm^2
      settings: SourceProductBaseCode=PW,SS,VE  InternalSimscapePortConfiguration="{\"Bottom\":[],\"Left\":[{\"id\":\"A\",\"label\":\"A\",\"type\":\"foundation.thermal_liquid.thermal_liquid\"}],\"Right\":[{\"id\":\"B\",\"label\":\"B\",\"type\":\"foundation.thermal_liquid.thermal_liquid\"}],\"Top\":[]}"
  Sensing Inlet Temperature : Subsystem
      mask Display: disp('T');
  Sensing Temperature : Subsystem
      mask Display: disp('T')
  Thermal Liquid Settings (TL) : fl_lib/Thermal Liquid/Utilities/Thermal Liquid Settings (TL)  table_dimensions=0  T_TLU=T K  p_TLU=p Pa  p_atm=1 atm  pT_region_flag=0  T_min=273.16 K  T_max=373.16 K  p_min=0.1 bar  p_max=500 bar  T_min_1D=273.16 K  T_max_1D=373.16 K  p_min_1D=0.01 MPa  p_max_1D=50 MPa  pT_validity_TLU=ones(11, 12)  rho_parameterization_2D=1  rho_parameterization_1D=1  rho_TLU=rho kg/m^3  beta_TLU=beta Pa  alpha_TLU=alpha 1/K  rho_TLU_2=[999.7973, 999.8431, 1002.3216, 1004.8218, 1007.293, 1009.7358, 1012.1506, 1014.5379, 1016.8979, 1019.2311, 1021.538, 1023.8188; 999.6579, 999.7009, 1002.0303, 1004.382, 1006.7084, 1009.0101, 1011.2874, 1013.5407, 1015.7703, 1017.9766, 1020.1599, 1022.3206; 998.1632, 998.2045, 1000.4375, 1002.6924, 1004.9239, 1007.1324, 1009.3183, 1011.4819, 1013.6236, 1015.7438, 1017.8428, 1019.921; 995.6057, 995.6458, 997.81864, 1000.0128, 1002.1841, 1004.3332, 1006.4603, 1008.566, 1010.6505, 1012.7144, 1014.758, 1016.7815; 992.1724, 992.2119, 994.35133, 996.5113, 998.6484, 1000.7633, 1002.8563, 1004.928, 1006.9788, 1009.009, 1011.0192, 1013.0097; 988.02, 988.0299, 990.15684, 992.3035, 994.4268, 996.5273, 998.6056, 1000.6622, 1002.6976, 1004.7123, 1006.7067, 1008.6813; 983.18, 983.1901, 985.3217, 987.4721, 989.5983, 991.7008, 993.7803, 995.8374, 997.8726, 999.8864, 1001.8795, 1003.8522; 977.75, 977.7583, 979.9094, 982.0783, 984.2216, 986.34, 988.4343, 990.505, 992.5529, 994.5786, 996.5825, 998.5654; 971.77, 971.7836, 973.96734, 976.1678, 978.3409, 980.4876, 982.6087, 984.7049, 986.7768, 988.8254, 990.8511, 992.8545; 965.26, 965.3023, 967.53107, 969.7753, 971.9901, 974.1764, 976.3354, 978.4676, 980.5741, 982.6556, 984.7129, 986.7465; 958.62, 958.6315, 960.627, 962.9267, 965.1944, 967.4314, 969.6387, 971.8173, 973.9681, 976.0921, 978.19, 980.2628] kg/m^3  rho_ref_3=998.21 kg/m^3  T_ref_3=293.16 K  p_ref_3=0.101325 MPa  beta_const_3=2.1791 GPa  alpha_const_3=2.0691e-4 1/K  rho_TLU_4=[999.84; 999.7; 998.2; 995.65; 992.21; 988.03; 983.19; 977.76; 971.78; 965.3; 958.8] kg/m^3  beta_const_4=2.1791 GPa  p_ref_4=0.101325 MPa  rho_ref_5=998.21 kg/m^3  T_ref_5=293.16 K  p_ref_5=0.101325 MPa  beta_const_5=2.1791 GPa  alpha_const_5=2.0691e-4 1/K  u_parameterization_2D=1  u_parameterization_1D=1  u_TLU=u J/g  cp_TLU=Cp J/K/g  u_TLU_2=[.0002, .0018, .086, .1588, .219, .267, .3034, .3288, .3436, .3483, .3435, .3294; 42.062, 42.06, 41.935, 41.804, 41.668, 41.527, 41.382, 41.233, 41.081, 40.924, 40.763, 40.599; 83.953, 83.948, 83.651, 83.349, 83.049, 82.749, 82.451, 82.153, 81.856, 81.56, 81.265, 80.971; 125.77, 125.76, 125.31, 124.86, 124.41, 123.97, 123.53, 123.1, 122.68, 122.25, 121.84, 121.42; 167.57, 167.56, 166.96, 166.37, 165.79, 165.21, 164.65, 164.09, 163.54, 163, 162.46, 161.94; 209.36, 209.36, 208.63, 207.9, 207.19, 206.48, 205.79, 205.11, 204.45, 203.79, 203.14, 202.5; 251.19, 251.19, 250.33, 249.47, 248.62, 247.79, 246.98, 246.18, 245.39, 244.62, 243.86, 243.12; 293.06, 293.06, 292.07, 291.07, 290.1, 289.14, 288.2, 287.28, 286.38, 285.49, 284.62, 283.77; 334.99, 334.99, 333.86, 332.73, 331.63, 330.54, 329.48, 328.44, 327.41, 326.41, 325.43, 324.46; 377, 377, 375.73, 374.46, 373.22, 372, 370.81, 369.64, 368.5, 367.38, 366.27, 365.19; 419.01, 419.01, 417.69, 416.27, 414.89, 413.54, 412.21, 410.91, 409.64, 408.4, 407.17, 405.98] kJ/kg  cp_TLU_3=[4.2199, 4.2194, 4.1957, 4.1726, 4.1508, 4.13, 4.1103, 4.0916, 4.0738, 4.0569, 4.0408, 4.0254; 4.1955, 4.1951, 4.1769, 4.1592, 4.1422, 4.1259, 4.1103, 4.0954, 4.0812, 4.0676, 4.0545, 4.0421; 4.1843, 4.184, 4.169, 4.1543, 4.1401, 4.1264, 4.1133, 4.1007, 4.0885, 4.0768, 4.0656, 4.0548; 4.1801, 4.1798, 4.1667, 4.1538, 4.1413, 4.1293, 4.1177, 4.1064, 4.0956, 4.0851, 4.075, 4.0653; 4.1796, 4.1794, 4.1675, 4.1558, 4.1444, 4.1334, 4.1227, 4.1123, 4.1023, 4.0926, 4.0832, 4.0741; 4.1813, 4.1813, 4.1702, 4.1592, 4.1484, 4.138, 4.1279, 4.1181, 4.1086, 4.0993, 4.0903, 4.0816; 4.185, 4.185, 4.1742, 4.1636, 4.1532, 4.1432, 4.1334, 4.1239, 4.1146, 4.1056, 4.0969, 4.0884; 4.1901, 4.1901, 4.1795, 4.169, 4.1588, 4.1489, 4.1393, 4.1299, 4.1207, 4.1118, 4.1032, 4.0947; 4.1968, 4.1968, 4.1862, 4.1757, 4.1655, 4.1555, 4.1458, 4.1364, 4.1273, 4.1183, 4.1096, 4.1012; 4.2052, 4.2052, 4.1944, 4.1837, 4.1733, 4.1632, 4.1534, 4.1438, 4.1345, 4.1255, 4.1166, 4.108; 4.2136, 4.2136, 4.2045, 4.1935, 4.1828, 4.1724, 4.1623, 4.1524, 4.1429, 4.1335, 4.1245, 4.1157] kJ/kg/K  u_TLU_4=[.0018; 42.06; 83.948; 125.76; 167.56; 209.36; 251.19; 293.06; 334.99; 377; 418.01] kJ/kg  cp_TLU_5=[4.2199; 4.1955; 4.1843; 4.1801; 4.1796; 4.1813; 4.185; 4.1901; 4.1968; 4.2052; 4.2136] kJ/kg/K  nu_TLU=nu cm^2/s  nu_TLU_2=[1.7917; 1.3061; 1.0032; .8006; .6577; .553; .4739; .4127; .3643; .3254; .2866] mm^2/s  k_TLU=k mW/m/K  k_TLU_2=[561.04; 580.02; 598.44; 615.48; 630.6; 643.61; 654.39; 663.13; 670.02; 675.27; 680.52] mW/m/K
      settings: SourceProductBaseCode=PW,SS,VE
  H1 : PMIOPort  Side=Left
  H2 : PMIOPort  Port=2  Side=Right
  connections:
  PS Terminator/LConn1 -- " Heat Exchanger Characteristic"/RConn3
  Sensing Temperature/RConn1 -- " Heat Exchanger Characteristic"/LConn3
  " Heat Exchanger Characteristic"/LConn1 -- Hose Radiator/LConn2
  Hose Radiator/LConn1 -- " Heat Exchanger Characteristic"/LConn2
  Hose Inlet/LConn1 -- Hose Radiator/RConn1 -- Sensing Temperature/LConn1
  Hose Outlet/LConn1 -- " Heat Exchanger Characteristic"/RConn2
  Pump/LConn1 -- Hose Outlet/RConn1 -- Thermal Liquid Settings (TL)/RConn1
  H2/RConn1 -- Convection Battery-Env/LConn1 -- " Heat Exchanger Characteristic"/RConn1
  Insulator Inlet Hose/LConn1 -- Hose Inlet/LConn2
  Insulator Outlet Hose/LConn1 -- Hose Outlet/LConn2
  Pipe/RConn1 -- Pump/RConn1 -- Sensing Inlet Temperature/LConn1
  Heat Exchanger Characteristic/LConn1 -- Pipe/LConn2
  Heat Exchanger Characteristic/RConn1 -- Convection Battery-Env/RConn1 -- H1/RConn1
  Pipe/LConn1 -- Heat Exchanger Characteristic/LConn2
  Heat Exchanger Characteristic/LConn3 -- Sensing Inlet Temperature/RConn1
  Expansion Tank/LConn1 -- Hose Inlet/RConn1 -- Heat Exchanger Characteristic/RConn2

== system ssc_auto_ev_20b/Step 2: Multirate Model/Driver and Environment ==
  Bus : Subsystem
  Bus Creator : BusCreator  Inputs=5
  Inclinometer : Subsystem
  Inputs : SignalEditorBlockLib/Signal Editor  FileName=ssc_auto_ev_Inputs.mat  ActiveScenario=Test_1  ActiveSignal=Env (deg C)  IsBus=off  OutputBusObjectStr=Bus: BusObject  SampleTime=0.01  OutputAfterFinalValue=Extrapolation  Unit=inherit  PreserveSignalName=on
  ZOH/{2..3,5..7} (5 alike) : ZeroOrderHold  SampleTime=dt
  Veh : Outport
  ECU : Outport  Port=2
  Env : Outport  Port=3
  wires:
  Inputs/2 -> Bus/2(Wi)
  Inclinometer/1(y) -> ZOH/6/1
  Inputs/4 -> ZOH/2/1
  Inputs/5 -> ZOH/3/1
  Inputs/1 -> Bus/1(In), Inclinometer/1(a)
  Inputs/6 -> ZOH/7/1
  Inputs/7 -> Env/1
  Bus/1(b) -> Veh/1
  Bus Creator/1 -> ECU/1
  ZOH/5/1 -> Bus Creator/2  "Brake pedal"
  ZOH/2/1 -> Bus Creator/3  "Throttle"
  ZOH/3/1 -> Bus Creator/4  "Cruise enable"
  ZOH/7/1 -> Bus Creator/5  "Cruise disable"
  ZOH/6/1 -> Bus Creator/1  "Incline"
  Inputs/3 -> ZOH/5/1, Bus/3(Br)

== system ssc_auto_ev_20b/Step 2: Multirate Model/Environment ==
  T : Inport
  Ambient Temperature : fl_lib/Thermal/Thermal Sources/Controlled Temperature Source
      settings: SourceProductBaseCode=PW,SS,VE
  Simulink-PS Converter1 : nesl_utility/Simulink-PS Converter  PhysicalDomain=network_engine_domain  SubClassName=ps_input  LeftPortType=input  RightPortType=output  PseudoPeriodic=off  Frequencies=[]  NoiseDistribution=none  NoiseParameters=[]  Unit=degC  AffineConversion=on  FilteringAndDerivatives=zero  SimscapeFilterOrder=1  InputFilterTimeConstant=.001  UdotUserProvided=1
      settings: SourceProductBaseCode=SS,PW,VE
  ThRef1 : fl_lib/Thermal/Thermal Elements/Thermal Reference
      settings: SourceProductBaseCode=PW,SS,VE
  E : PMIOPort  Side=Right
  wires:
  T/1 -> Simulink-PS Converter1/1
  connections:
  Ambient Temperature/RConn2 -- ThRef1/LConn1
  Ambient Temperature/RConn1 -- Simulink-PS Converter1/RConn1
  Ambient Temperature/LConn1 -- E/RConn1
